simulink model "ADRC_22_TEST"  (Simulink 7.6)
settings: Solver=ode45  StartTime=0.0  StopTime=500  RelTol=1e-3
libraries: ADRC x2
settings Model: Creator=Administrator  LastModifiedBy=Administrator
settings DebuggingCC: AlgebraicLoopMsg=none  ArtificialAlgebraicLoopMsg=none  SolverPrmCheckMsg=none  UnknownTsInhSupMsg=none

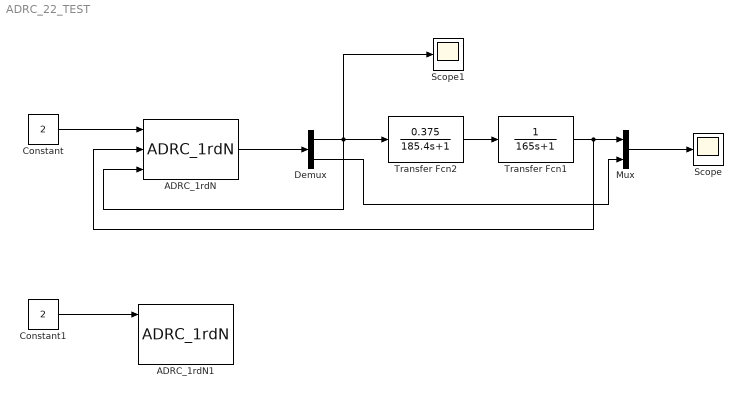
== system ADRC_22_TEST ==
  ADRC_1rdN : ADRC/ADRC/ADRC_1rd/ADRC_1rdN  SystemSampleTime=-1  RT=300  h=0.05  B01=20  B02=100  r=0.01
  ADRC_1rdN1 : ADRC/ADRC/ADRC_1rd/ADRC_1rdN  SystemSampleTime=-1  RT=300  h=0.05  B01=20  B02=100  r=0.01
  Constant : Constant  Value=2
  Constant1 : Constant  Value=2
  Demux : Demux  Outputs=2
  Mux : Mux  Inputs=2
  Scope : Scope
      settings: TimeRange=200  YMin=3  YMax=11.5  DataFormat=Array
  Scope1 : Scope
      settings: TimeRange=50  YMin=0  YMax=250  DataFormat=Array
  Transfer Fcn1 : TransferFcn  Numerator=1  Denominator=[165 1]
  Transfer Fcn2 : TransferFcn  Numerator=0.375  Denominator=[185.4 1]
  wires:
  Constant/1 -> ADRC_1rdN/1
  Transfer Fcn2/1 -> Transfer Fcn1/1
  ADRC_1rdN/1 -> Demux/1
  Demux/1 -> Transfer Fcn2/1, ADRC_1rdN/3, Scope1/1
  Transfer Fcn1/1 -> Mux/1, ADRC_1rdN/2
  Demux/2 -> Mux/2
  Mux/1 -> Scope/1
  Constant1/1 -> ADRC_1rdN1/1
